simulink model "rtwdemo_srbb"  (Simulink 6.0)
settings: Solver=FixedStepDiscrete  StartTime=0.0  StopTime=10.0  RelTol=1e-3  SampleTimeConstraint=Specified
undefined symbols (not defined in the file or in its folder): DiscIntNeverNeededParam
libraries: rtwdemowidgets x3
settings Model: Creator=The MathWorks Inc.  LastModifiedBy=batserve  ExtModeArmWhenConnect=off  ExtModeAutoUpdateStatusClock=off
settings MATStruct: SampleTime=1  Offset=0  Priority=[0.0]
settings DataIOCC: SaveOutput=off  SaveTime=off  SignalLoggingName=sigsOut
settings OptimizationCC: InlineParams=on  EnforceIntegerDowncast=off  StateBitsets=on  DataBitsets=on  UseTempVars=on
settings DebuggingCC: CheckExecutionContextPreStartOutputMsg=on  CheckExecutionContextRuntimeOutputMsg=on  SolverPrmCheckMsg=none  UnconnectedInputMsg=none  UnconnectedOutputMsg=none  UnconnectedLineMsg=none
settings ModelReferenceCC: UpdateModelReferenceTargets=IfOutOfDate
settings RTWCC: TLCOptions=-p0 -aWarnNonSaturatedBlocks=0  GenerateReport=on  RTWVerbose=off  ProcessScript=grt_make_rtw_hook  LaunchReport=on
settings CodeAppCC: ForceParamTrailComments=on  PrefixModelToSubsysFcnNames=off
settings GRTTargetCC: MatFileLogging=off

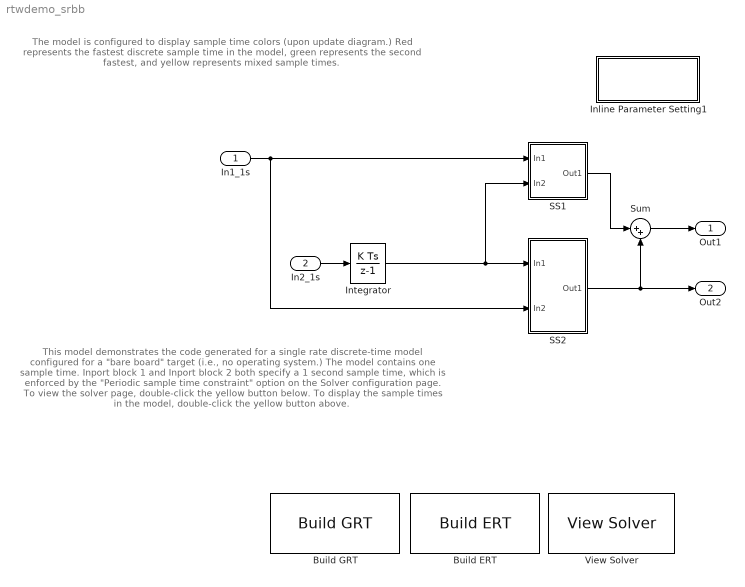
== system rtwdemo_srbb ==
  note: This model demonstrates the code generated for a single rate discrete-time model
      | configured for a "bare board" target (i.e., no operating system.)  The model contains
      | one sample time.  Inport block 1 and Inport block 2 both specify a 1 second sample
      | time, which is enforced by the "Periodic sample time constraint" option on the Solver
      | configuration page.  To view the solver page, double-click the yellow button below.
      | To display the sample times in the model, double-click the yellow button above.
  note: The model is configured to display sample time colors (upon
      | update diagram.)  Red represents the fastest discrete sample
      | time in the model, green represents the second fastest,
      | and yellow represents mixed sample times.
  In1_1s : Inport  Port=1  SampleTime=1  LatchInput=off
  In2_1s : Inport  Port=2  SampleTime=1  LatchInput=off
  Build ERT : rtwdemowidgets/Build ERT  attrib_overrides={}
  Build GRT : rtwdemowidgets/Build GRT  attrib_overrides={}
  Inline Parameter Setting1 : Subsystem  Orientation=up  PropExecContextAcrossSSBoundary=on
      settings: OpenFcn=m=get_param(bdroot,'name'); eval([m,'([],[],[],''compile'');']); eval([m,'([],[],[],''term'');']);
      mask Display: disp(sprintf('Display Sample\nTime Colors\n(double-click)'))
  Integrator : DiscreteIntegrator  InitialConditionMode=State only (most efficient)  SampleTime=-1  SaturateOnIntegerOverflow=on  ICPrevOutput=DiscIntNeverNeededParam  ICPrevScaledInput=DiscIntNeverNeededParam
  SS1 : Subsystem  TreatAsAtomicUnit=on  PropExecContextAcrossSSBoundary=on
  SS2 : Subsystem  TreatAsAtomicUnit=on  PropExecContextAcrossSSBoundary=on
  Sum : Sum  Inputs=|++  SaturateOnIntegerOverflow=on  InputSameDT=on
  View Solver : rtwdemowidgets/View Solver
  Out1 : Outport
  Out2 : Outport  Port=2
  wires:
  In1_1s/1 -> SS1/1(In1), SS2/2(In2)
  In2_1s/1 -> Integrator/1
  SS2/1(Out1) -> Out2/1, Sum/2
  SS1/1(Out1) -> Sum/1
  Sum/1 -> Out1/1
  Integrator/1 -> SS2/1(In1), SS1/2(In2)

== system rtwdemo_srbb/Inline Parameter Setting1 ==

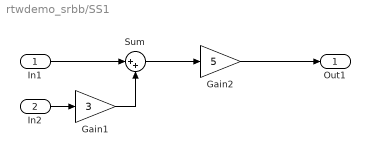
== system rtwdemo_srbb/SS1 ==
  In1 : Inport  Port=1  LatchInput=off
  In2 : Inport  Port=2  LatchInput=off
  Gain1 : Gain  Gain=3  SaturateOnIntegerOverflow=on
  Gain2 : Gain  Gain=5  SaturateOnIntegerOverflow=on
  Sum : Sum  Inputs=|++  SaturateOnIntegerOverflow=on  InputSameDT=on
  Out1 : Outport
  wires:
  In1/1 -> Sum/1
  Sum/1 -> Gain2/1
  In2/1 -> Gain1/1
  Gain2/1 -> Out1/1
  Gain1/1 -> Sum/2

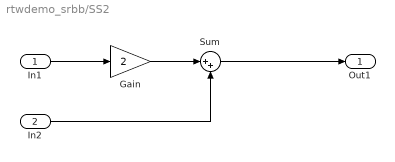
== system rtwdemo_srbb/SS2 ==
  In1 : Inport  Port=1  LatchInput=off
  In2 : Inport  Port=2  LatchInput=off
  Gain : Gain  Gain=2  SaturateOnIntegerOverflow=on
  Sum : Sum  Inputs=|++  SaturateOnIntegerOverflow=on  InputSameDT=on
  Out1 : Outport
  wires:
  In1/1 -> Gain/1
  Gain/1 -> Sum/1
  Sum/1 -> Out1/1
  In2/1 -> Sum/2
